simulink model "SSIV_Simulink_Com2"  (R2018a)
settings: Solver=FixedStepAuto  StartTime=0.0  StopTime=inf  FixedStep=.015  RelTol=1e-3  EnableMultiTasking=on
libraries: hdlsllib x51, raspberrypilib x16, simulink x10
(part 1 of 2)
settings Model: SimulationMode=external  Creator=domin  LastModifiedBy=cbirdson
settings SolverCC: ConcurrentTasks=on  PositivePriorityOrder=on  AutoInsertRateTranBlk=on
settings DataIOCC: SaveFormat=Array
settings OptimizationCC: EnhancedBackFolding=on  PassReuseOutputArgsThreshold=0  MaxStackSize=64  OptimizeBlockOrder=speed  DifferentSizesBufferReuse=on  OptimizationCustomize=off
settings DebuggingCC: ParameterTunabilityLossMsg=error
settings HardwareCC: ProdBitPerPointer=32  ProdBitPerSizeT=32  ProdBitPerPtrDiffT=32  ProdLargestAtomicInteger=Long  ProdLargestAtomicFloat=Double  ProdWordSize=32  ProdHWDeviceType=ARM Compatible->ARM Cortex  UseEmbeddedCoderFeatures=off  UseSimulinkCoderFeatures=off
settings SFSimCC: MATLABDynamicMemAlloc=off
settings RTWCC: SystemTargetFile=ert.tlc  HardwareBoard=Raspberry Pi  TLCOptions="-aInlineSetEventsForThisBaseRateFcn=TLC_FALSE -aSuppressMultiTaskScheduler=TLC_FALSE  -aRateBasedStepFcn=0"  TemplateMakefile=ert_default_tmf  RTWVerbose=off  Toolchain=GNU GCC Raspberry Pi  BuildConfiguration=Faster Runs
settings CodeAppCC: ForceParamTrailComments=on  OperatorAnnotations=on  MangleLength=10
settings ERTTargetCC: ERTCustomFileBanners=off  SupportContinuousTime=on  SupportNonInlinedSFcns=on  RemoveResetFunc=off  SupportVariableSizeSignals=on  ModelStepFunctionPrototypeControlCompliant=off  ExtMode=on  ExtModeMexArgs='129.65.101.12' 0 17725  ERTSrcFileBannerTemplate=codertarget_code_template.cgt  ERTHdrFileBannerTemplate=codertarget_code_template.cgt  ERTDataSrcFileTemplate=codertarget_code_template.cgt  ERTDataHdrFileTemplate=codertarget_code_template.cgt

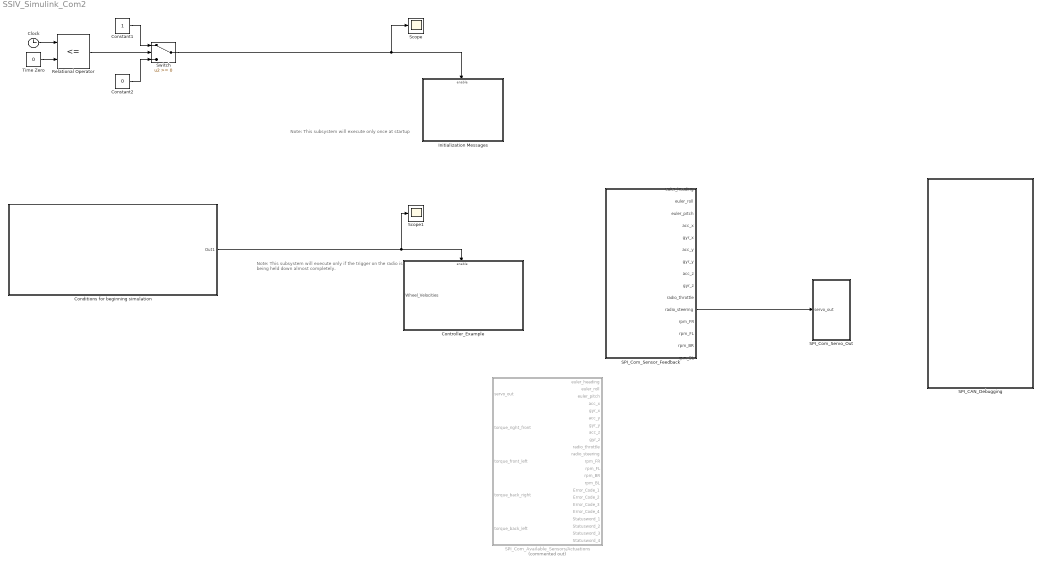
== system SSIV_Simulink_Com2 ==
  note: Note: This subsystem will execute only once at startup
  note: Note: This subsystem will execute only if the trigger on the radio
      | is being held down almost completely.
  Clock : Clock
  Conditions for beginning simulation : Subsystem
  Constant1 : Constant
  Constant2 : Constant  Value=0
  Controller_Example : Subsystem
  Initialization Messages : Subsystem
  Relational Operator : RelationalOperator  Operator=<=  OutDataTypeStr=boolean  RndMeth=Simplest
  SPI_CAN_Debugging : Subsystem
  SPI_Com_Available_Sensors/Actuations : Subsystem  Commented=on
  SPI_Com_Sensor_Feedback : Subsystem
  SPI_Com_Servo_Out : Subsystem
  Scope : Scope
  Scope1 : Scope
  Switch : Switch
  Time Zero : Constant  Value=0
  wires:
  Relational Operator/1 -> Switch/2
  Time Zero/1 -> Relational Operator/2
  Constant2/1 -> Switch/3
  Clock/1 -> Relational Operator/1
  Switch/1 -> Initialization Messages/Enable, Scope/1
  Constant1/1 -> Switch/1
  Conditions for beginning simulation/1(Out1) -> Controller_Example/Enable, Scope1/1
  SPI_Com_Sensor_Feedback/11(radio_steering) -> SPI_Com_Servo_Out/1(servo_out)

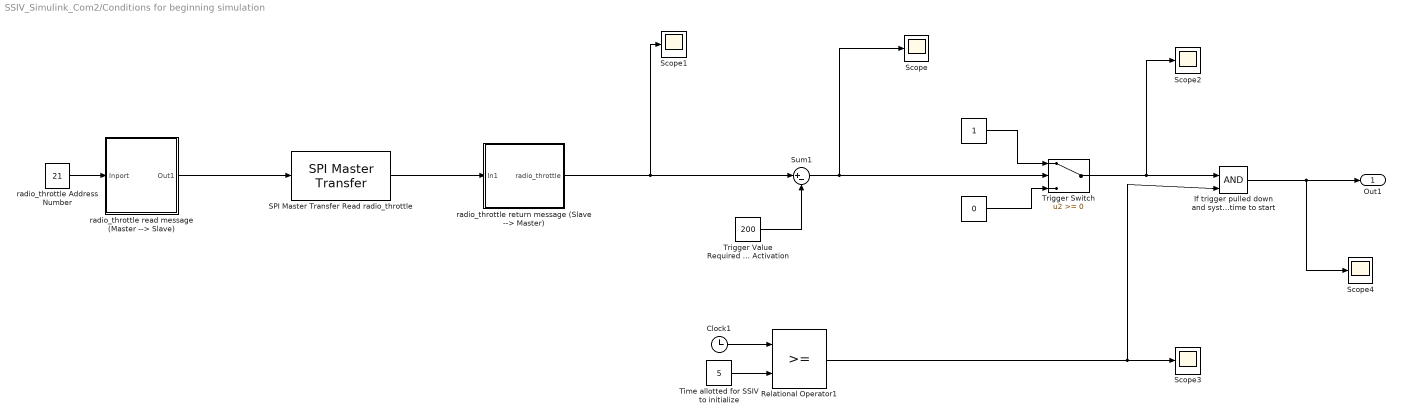
== system SSIV_Simulink_Com2/Conditions for beginning simulation ==
  " " : Constant  Value=0
  "   " : Constant
  Clock1 : Clock
  If trigger pulled down and system given enough time to start : Logic  IconShape=distinctive  AllPortsSameDT=off  OutDataTypeStr=boolean
  Relational Operator1 : RelationalOperator  OutDataTypeStr=boolean  RndMeth=Simplest
  SPI Master Transfer Read radio_throttle : raspberrypilib/SPI Master Transfer  BoardProperty=Pi 3 Model B  SPIModule=uint32(0)  Mode=Master  BusSpeed=1000000  Pin=SPI0_CE1  FirstBitToTransfer=Most significant bit (MSB)  ClockMode=0  BlockFunction=Transfer  RegisterAddress=0  OutputDataType=int8  OutputDataLength=1
      settings: SourceProductName=Simulink Support Package for Raspberry Pi Hardware  SourceProductBaseCode=RASPPI
  Scope{,1..4} (5 alike) : Scope
  Sum1 : Sum  Inputs=|+-
  Time allotted for SSIV to initialize : Constant  Value=5
  Trigger Switch : Switch
  Trigger Value Required for Subsystem Activation : Constant  Value=200
  "radio_throttle Address Number " : Constant  Value=21  OutDataTypeStr=uint8
  radio_throttle read message (Master --> Slave) : Subsystem
  radio_throttle return message (Slave --> Master) : Subsystem
  Out1 : Outport
  wires:
  " "/1 -> Trigger Switch/3
  Trigger Switch/1 -> Scope2/1, If trigger pulled down and system given enough time to start/1
  SPI Master Transfer Read radio_throttle/1 -> radio_throttle return message (Slave --> Master)/1(In1)
  Time allotted for SSIV to initialize/1 -> Relational Operator1/2
  "radio_throttle Address Number "/1 -> radio_throttle read message (Master --> Slave)/1(Inport)
  Clock1/1 -> Relational Operator1/1
  Relational Operator1/1 -> Scope3/1, If trigger pulled down and system given enough time to start/2
  Sum1/1 -> Scope/1, Trigger Switch/2
  radio_throttle read message (Master --> Slave)/1(Out1) -> SPI Master Transfer Read radio_throttle/1
  Trigger Value Required for Subsystem Activation/1 -> Sum1/2
  "   "/1 -> Trigger Switch/1
  If trigger pulled down and system given enough time to start/1 -> Scope4/1, Out1/1
  radio_throttle return message (Slave --> Master)/1(radio_throttle) -> Scope1/1, Sum1/1

== system SSIV_Simulink_Com2/Controller_Example ==
  "Wheel_Velocities " : Inport
  Enable : EnablePort
  Const Mot Torque mNm : Constant  Value=100
  Const Mot Torque mNm1 : Constant  Value=100
  Gain : Gain
  Gain1 : Gain
  SPI_Communication_Torque_Actuations : Subsystem
  wires:
  Const Mot Torque mNm/1 -> Gain/1
  Const Mot Torque mNm1/1 -> Gain1/1
  Gain/1 -> SPI_Communication_Torque_Actuations/2(torque_front_left), SPI_Communication_Torque_Actuations/1(torque_right_front)
  Gain1/1 -> SPI_Communication_Torque_Actuations/4(torque_back_left), SPI_Communication_Torque_Actuations/3(torque_back_right)

== system SSIV_Simulink_Com2/Initialization Messages ==
  Enable : EnablePort
  Dead Switch : Constant  OutDataTypeStr=uint8
  Display3 : Display
      settings: Format=decimal (Stored Integer)
  Display4 : Display
      settings: Format=decimal (Stored Integer)
  Display5 : Display
      settings: Format=decimal (Stored Integer)
  IMU Reset : Constant  OutDataTypeStr=uint8
  Initialize Motor Controllers Command : Constant  OutDataTypeStr=uint8
  SPI Register Write dead_switch : raspberrypilib/SPI Register Write  BoardProperty=Pi 3 Model B  SPIModule=uint32(0)  Mode=Master  BusSpeed=1000000  Pin=SPI0_CE1  FirstBitToTransfer=Most significant bit (MSB)  ClockMode=0  BlockFunction=Write  RegisterAddress=2  OutputDataType=int8  OutputDataLength=1
      settings: SourceProductName=Simulink Support Package for Raspberry Pi Hardware  SourceProductBaseCode=RASPPI
  SPI Register Write init_motor_controllers : raspberrypilib/SPI Register Write  BoardProperty=Pi 3 Model B  SPIModule=uint32(0)  Mode=Master  BusSpeed=1000000  Pin=SPI0_CE1  FirstBitToTransfer=Most significant bit (MSB)  ClockMode=0  BlockFunction=Write  RegisterAddress=0  OutputDataType=int8  OutputDataLength=1
      settings: SourceProductName=Simulink Support Package for Raspberry Pi Hardware  SourceProductBaseCode=RASPPI
  SPI Register Write reset_imu : raspberrypilib/SPI Register Write  BoardProperty=Pi 3 Model B  SPIModule=uint32(0)  Mode=Master  BusSpeed=1000000  Pin=SPI0_CE1  FirstBitToTransfer=Most significant bit (MSB)  ClockMode=0  BlockFunction=Write  RegisterAddress=1  OutputDataType=int8  OutputDataLength=1
      settings: SourceProductName=Simulink Support Package for Raspberry Pi Hardware  SourceProductBaseCode=RASPPI
  wires:
  Initialize Motor Controllers Command/1 -> Display3/1, SPI Register Write init_motor_controllers/1
  IMU Reset/1 -> SPI Register Write reset_imu/1, Display4/1
  Dead Switch/1 -> Display5/1, SPI Register Write dead_switch/1

== system SSIV_Simulink_Com2/SPI_CAN_Debugging ==
  Bitwise AND : simulink/Logic and Bit Operations/Bitwise Operator  logicop=AND  UseBitMask=on  BitMask=bin2dec('01101111')  BitMaskRealWorld=Stored Integer
  Debugging : Scope  NumInputPorts=2
  ERROR_REGISTERS : Display
      settings: Format=binary (Stored Integer)
  Error and Statusword read message (Master --> Slave) : Subsystem
  Errors and Statuswords return message (Slave --> Master) : Subsystem
  Mux : Mux
  Mux1 : Mux
  SPI Master Transfer Read Errors and Statuswords : raspberrypilib/SPI Master Transfer  BoardProperty=Pi 3 Model B  SPIModule=uint32(0)  Mode=Master  BusSpeed=1000000  Pin=SPI0_CE1  FirstBitToTransfer=Most significant bit (MSB)  ClockMode=0  BlockFunction=Transfer  RegisterAddress=0  OutputDataType=int8  OutputDataLength=1
      settings: SourceProductName=Simulink Support Package for Raspberry Pi Hardware  SourceProductBaseCode=RASPPI
  STATUSWORDS : Display
      settings: Format=binary (Stored Integer)
  node_errors[0] Address Number : Constant  Value=44  OutDataTypeStr=uint8
  wires:
  Error and Statusword read message (Master --> Slave)/1(Out1) -> SPI Master Transfer Read Errors and Statuswords/1
  node_errors[0] Address Number/1 -> Error and Statusword read message (Master --> Slave)/1(Inport)
  SPI Master Transfer Read Errors and Statuswords/1 -> Bitwise AND/1
  Bitwise AND/1 -> Errors and Statuswords return message (Slave --> Master)/1(In1)
  Errors and Statuswords return message (Slave --> Master)/1(Error_Code_1) -> Mux/1
  Errors and Statuswords return message (Slave --> Master)/2(Error_Code_2) -> Mux/2
  Errors and Statuswords return message (Slave --> Master)/3(Error_Code_3) -> Mux/3
  Errors and Statuswords return message (Slave --> Master)/4(Error_Code_4) -> Mux/4
  Mux/1 -> ERROR_REGISTERS/1, Debugging/1
  Errors and Statuswords return message (Slave --> Master)/5(Statusword_1) -> Mux1/1
  Errors and Statuswords return message (Slave --> Master)/6(Statusword_2) -> Mux1/2
  Errors and Statuswords return message (Slave --> Master)/7(Statusword_3) -> Mux1/3
  Errors and Statuswords return message (Slave --> Master)/8(Statusword_4) -> Mux1/4
  Mux1/1 -> STATUSWORDS/1, Debugging/2

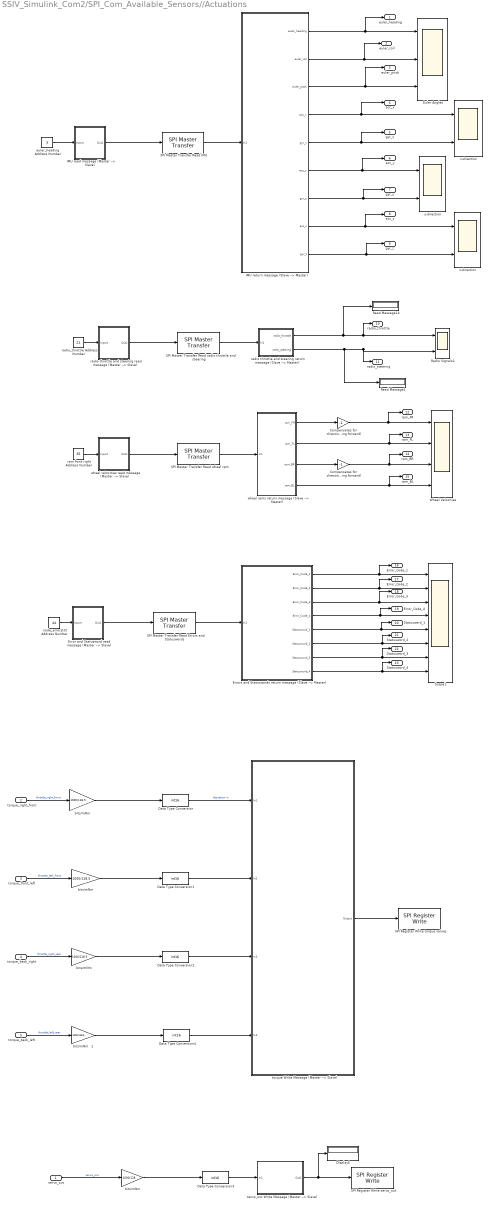
== system SSIV_Simulink_Com2/SPI_Com_Available_Sensors//Actuations ==
  servo_out : Inport
  torque_right_front : Inport  Port=2
  torque_front_left : Inport  Port=3
  torque_back_right : Inport  Port=4
  torque_back_left : Inport  Port=5
  Compensates for direction of spin (want positive to be rolling forward) : Gain  Gain=-1
  "Compensates for direction of spin (want positive to be rolling forward)  " : Gain  Gain=-1
  Data Type Conversion{,1..4} (5 alike) : DataTypeConversion  OutDataTypeStr=int16  RndMeth=Nearest
  Display5 : Display
      settings: Format=decimal (Stored Integer)
  Error and Statusword read message (Master --> Slave) : Subsystem
  Errors and Statuswords return message (Slave --> Master) : Subsystem
  Euler Angles : Scope  NumInputPorts=3
  IMU read message (Master --> Slave) : Subsystem
  IMU return message (Slave --> Master) : Subsystem
  Radio SIgnals2 : Scope  NumInputPorts=2
  Read Message1 : Display
      settings: Format=decimal (Stored Integer)
  Read Message14 : Display
      settings: Format=decimal (Stored Integer)
  SPI Master Transfer Read Errors and Statuswords : raspberrypilib/SPI Master Transfer  BoardProperty=Pi 3 Model B  SPIModule=uint32(0)  Mode=Master  BusSpeed=1000000  Pin=SPI0_CE1  FirstBitToTransfer=Most significant bit (MSB)  ClockMode=0  BlockFunction=Transfer  RegisterAddress=0  OutputDataType=int8  OutputDataLength=1
      settings: SourceProductName=Simulink Support Package for Raspberry Pi Hardware  SourceProductBaseCode=RASPPI
  SPI Master Transfer Read IMU : raspberrypilib/SPI Master Transfer  BoardProperty=Pi 3 Model B  SPIModule=uint32(0)  Mode=Master  BusSpeed=1000000  Pin=SPI0_CE1  FirstBitToTransfer=Most significant bit (MSB)  ClockMode=0  BlockFunction=Transfer  RegisterAddress=0  OutputDataType=int8  OutputDataLength=1
      settings: SourceProductName=Simulink Support Package for Raspberry Pi Hardware  SourceProductBaseCode=RASPPI
  SPI Master Transfer Read radio throttle and steering : raspberrypilib/SPI Master Transfer  BoardProperty=Pi 3 Model B  SPIModule=uint32(0)  Mode=Master  BusSpeed=1000000  Pin=SPI0_CE1  FirstBitToTransfer=Most significant bit (MSB)  ClockMode=0  BlockFunction=Transfer  RegisterAddress=0  OutputDataType=int8  OutputDataLength=1
      settings: SourceProductName=Simulink Support Package for Raspberry Pi Hardware  SourceProductBaseCode=RASPPI
  SPI Master Transfer Read wheel rpm : raspberrypilib/SPI Master Transfer  BoardProperty=Pi 3 Model B  SPIModule=uint32(0)  Mode=Master  BusSpeed=1000000  Pin=SPI0_CE1  FirstBitToTransfer=Most significant bit (MSB)  ClockMode=0  BlockFunction=Transfer  RegisterAddress=0  OutputDataType=int8  OutputDataLength=1
      settings: SourceProductName=Simulink Support Package for Raspberry Pi Hardware  SourceProductBaseCode=RASPPI
  "SPI Register Write servo_out " : raspberrypilib/SPI Register Write  BoardProperty=Pi 3 Model B  SPIModule=uint32(0)  Mode=Master  BusSpeed=1000000  Pin=SPI0_CE1  FirstBitToTransfer=Most significant bit (MSB)  ClockMode=0  BlockFunction=Write  RegisterAddress=33  OutputDataType=int8  OutputDataLength=1
      settings: SourceProductName=Simulink Support Package for Raspberry Pi Hardware  SourceProductBaseCode=RASPPI
  SPI Register Write torque values : raspberrypilib/SPI Register Write  BoardProperty=Pi 3 Model B  SPIModule=uint32(0)  Mode=Master  BusSpeed=1000000  Pin=SPI0_CE1  FirstBitToTransfer=Most significant bit (MSB)  ClockMode=0  BlockFunction=Write  RegisterAddress=25  OutputDataType=int8  OutputDataLength=1
      settings: SourceProductName=Simulink Support Package for Raspberry Pi Hardware  SourceProductBaseCode=RASPPI
  Scope1 : Scope  NumInputPorts=8
  Wheel Velocities : Scope  NumInputPorts=4
  bits/mNm : Gain  Gain=1000/118.5
  "bits/mNm " : Gain  Gain=1000/118.5
  "bits/mNm  " : Gain  Gain=1000/118.5
  "bits/mNm    " : Gain  Gain=1000/128
  bits/mNm   1 : Gain  Gain=1000/118.5
  euler_heading Address Number : Constant  Value=3  OutDataTypeStr=uint8
  node_errors[0] Address Number : Constant  Value=44  OutDataTypeStr=uint8
  radio throttle and steering read message (Master --> Slave) : Subsystem
  radio throttle and steering return message (Slave --> Master) : Subsystem
  "radio_throttle Address Number " : Constant  Value=21  OutDataTypeStr=uint8
  "rpm front right Address Number " : Constant  Value=35  OutDataTypeStr=uint8
  servo_out Write Message (Master --> Slave) : Subsystem
  torque Write Message (Master --> Slave) : Subsystem
  wheel rpms return message (Slave --> Master) : Subsystem
  wheel velocities read message (Master --> Slave) : Subsystem
  x-direction : Scope  NumInputPorts=2
  y-direction : Scope  NumInputPorts=2
  z-direction : Scope  NumInputPorts=2
  euler_heading : Outport
  euler_roll : Outport  Port=2
  euler_pitch : Outport  Port=3
  acc_x : Outport  Port=4
  gyr_x : Outport  Port=5
  acc_y : Outport  Port=6
  gyr_y : Outport  Port=7
  acc_z : Outport  Port=8
  gyr_z : Outport  Port=9
  radio_throttle : Outport  Port=10
  radio_steering : Outport  Port=11
  rpm_FR : Outport  Port=12
  rpm_FL : Outport  Port=13
  rpm_BR : Outport  Port=14
  rpm_BL : Outport  Port=15
  Error_Code_1 : Outport  Port=16
  Error_Code_2 : Outport  Port=17
  Error_Code_3 : Outport  Port=18
  Error_Code_4 : Outport  Port=19
  Statusword_1 : Outport  Port=20
  Statusword_2 : Outport  Port=21
  Statusword_3 : Outport  Port=22
  Statusword_4 : Outport  Port=23
  wires:
  IMU read message (Master --> Slave)/1(Out1) -> SPI Master Transfer Read IMU/1
  SPI Master Transfer Read IMU/1 -> IMU return message (Slave --> Master)/1(In1)
  SPI Master Transfer Read wheel rpm/1 -> wheel rpms return message (Slave --> Master)/1(In1)
  wheel rpms return message (Slave --> Master)/1(rpm_FR) -> Compensates for direction of spin (want positive to be rolling forward)/1
  servo_out/1 -> "bits/mNm    "/1  "servo_out"
  servo_out Write Message (Master --> Slave)/1(Out1) -> Display5/1, "SPI Register Write servo_out "/1
  torque Write Message (Master --> Slave)/1(Output) -> SPI Register Write torque values/1
  Data Type Conversion/1 -> torque Write Message (Master --> Slave)/1(In1)  "Actuation in"
  Data Type Conversion1/1 -> torque Write Message (Master --> Slave)/2(In2)
  Data Type Conversion2/1 -> torque Write Message (Master --> Slave)/3(In3)
  Data Type Conversion3/1 -> servo_out Write Message (Master --> Slave)/1(In1)
  Data Type Conversion4/1 -> torque Write Message (Master --> Slave)/4(In4)
  euler_heading Address Number/1 -> IMU read message (Master --> Slave)/1(Inport)
  "radio_throttle Address Number "/1 -> radio throttle and steering read message (Master --> Slave)/1(Inport)
  radio throttle and steering return message (Slave --> Master)/1(radio_throttle) -> Radio SIgnals2/1, radio_throttle/1, Read Message14/1
  SPI Master Transfer Read radio throttle and steering/1 -> radio throttle and steering return message (Slave --> Master)/1(In1)
  radio throttle and steering read message (Master --> Slave)/1(Out1) -> SPI Master Transfer Read radio throttle and steering/1
  bits/mNm/1 -> Data Type Conversion/1
  "bits/mNm "/1 -> Data Type Conversion1/1
  "bits/mNm  "/1 -> Data Type Conversion2/1
  bits/mNm   1/1 -> Data Type Conversion4/1
  "bits/mNm    "/1 -> Data Type Conversion3/1
  Compensates for direction of spin (want positive to be rolling forward)/1 -> Wheel Velocities/1, rpm_FR/1
  Error and Statusword read message (Master --> Slave)/1(Out1) -> SPI Master Transfer Read Errors and Statuswords/1
  SPI Master Transfer Read Errors and Statuswords/1 -> Errors and Statuswords return message (Slave --> Master)/1(In1)
  node_errors[0] Address Number/1 -> Error and Statusword read message (Master --> Slave)/1(Inport)
  Errors and Statuswords return message (Slave --> Master)/1(Error_Code_1) -> Error_Code_1/1, Scope1/1
  Errors and Statuswords return message (Slave --> Master)/2(Error_Code_2) -> Error_Code_2/1, Scope1/2
  Errors and Statuswords return message (Slave --> Master)/3(Error_Code_3) -> Error_Code_3/1, Scope1/3
  Errors and Statuswords return message (Slave --> Master)/4(Error_Code_4) -> Error_Code_4/1, Scope1/4
  Errors and Statuswords return message (Slave --> Master)/5(Statusword_1) -> Statusword_1/1, Scope1/5
  Errors and Statuswords return message (Slave --> Master)/6(Statusword_2) -> Statusword_2/1, Scope1/6
  Errors and Statuswords return message (Slave --> Master)/7(Statusword_3) -> Statusword_3/1, Scope1/7
  Errors and Statuswords return message (Slave --> Master)/8(Statusword_4) -> Statusword_4/1, Scope1/8
  "rpm front right Address Number "/1 -> wheel velocities read message (Master --> Slave)/1(Inport)
  wheel velocities read message (Master --> Slave)/1(Out1) -> SPI Master Transfer Read wheel rpm/1
  wheel rpms return message (Slave --> Master)/2(rpm_FL) -> rpm_FL/1, Wheel Velocities/2
  wheel rpms return message (Slave --> Master)/3(rpm_BR) -> "Compensates for direction of spin (want positive to be rolling forward)  "/1
  "Compensates for direction of spin (want positive to be rolling forward)  "/1 -> rpm_BR/1, Wheel Velocities/3
  wheel rpms return message (Slave --> Master)/4(rpm_BL) -> rpm_BL/1, Wheel Velocities/4
  radio throttle and steering return message (Slave --> Master)/2(radio_steering) -> Read Message1/1, radio_steering/1, Radio SIgnals2/2
  IMU return message (Slave --> Master)/1(euler_heading) -> euler_heading/1, Euler Angles/1
  IMU return message (Slave --> Master)/2(euler_roll) -> euler_roll/1, Euler Angles/2
  IMU return message (Slave --> Master)/3(euler_pitch) -> euler_pitch/1, Euler Angles/3
  IMU return message (Slave --> Master)/4(acc_x) -> acc_x/1, x-direction/1
  IMU return message (Slave --> Master)/5(gyr_x) -> gyr_x/1, x-direction/2
  IMU return message (Slave --> Master)/6(acc_y) -> acc_y/1, y-direction/1
  IMU return message (Slave --> Master)/7(gyr_y) -> gyr_y/1, y-direction/2
  IMU return message (Slave --> Master)/8(acc_z) -> acc_z/1, z-direction/1
  IMU return message (Slave --> Master)/9(gyr_z) -> gyr_z/1, z-direction/2
  torque_back_left/1 -> bits/mNm   1/1  "throttle_left_rear"
  torque_right_front/1 -> bits/mNm/1  "throttle_right_front"
  torque_front_left/1 -> "bits/mNm "/1  "throttle_left_front"
  torque_back_right/1 -> "bits/mNm  "/1  "throttle_right_rear"

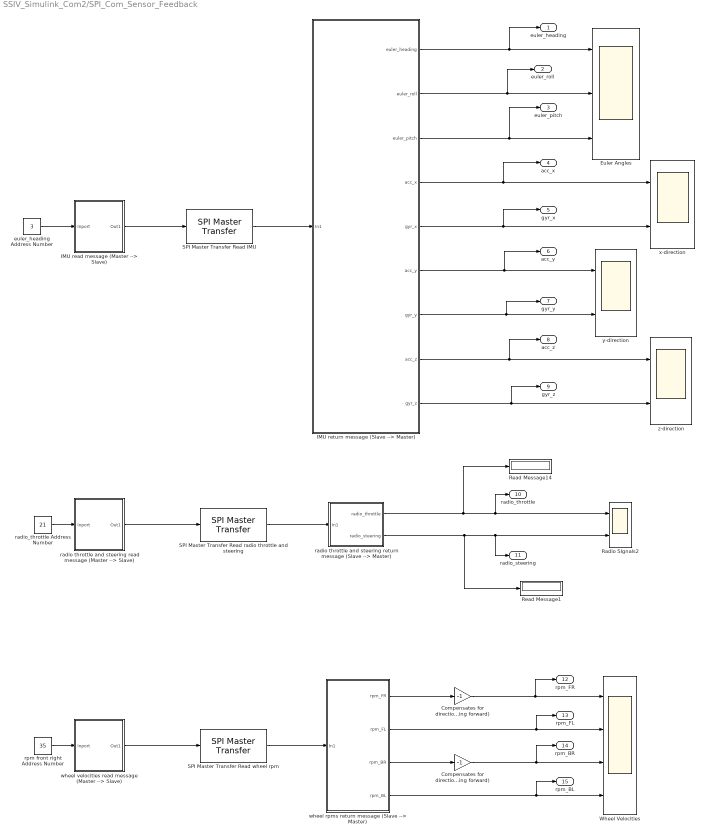
== system SSIV_Simulink_Com2/SPI_Com_Sensor_Feedback ==
  Compensates for direction of spin (want positive to be rolling forward) : Gain  Gain=-1
  "Compensates for direction of spin (want positive to be rolling forward)  " : Gain  Gain=-1
  Euler Angles : Scope  NumInputPorts=3
  IMU read message (Master --> Slave) : Subsystem
  IMU return message (Slave --> Master) : Subsystem
  Radio SIgnals2 : Scope  NumInputPorts=2
  Read Message1 : Display
      settings: Format=decimal (Stored Integer)
  Read Message14 : Display
      settings: Format=decimal (Stored Integer)
  SPI Master Transfer Read IMU : raspberrypilib/SPI Master Transfer  BoardProperty=Pi 3 Model B  SPIModule=uint32(0)  Mode=Master  BusSpeed=1000000  Pin=SPI0_CE1  FirstBitToTransfer=Most significant bit (MSB)  ClockMode=0  BlockFunction=Transfer  RegisterAddress=0  OutputDataType=int8  OutputDataLength=1
      settings: SourceProductName=Simulink Support Package for Raspberry Pi Hardware  SourceProductBaseCode=RASPPI
  SPI Master Transfer Read radio throttle and steering : raspberrypilib/SPI Master Transfer  BoardProperty=Pi 3 Model B  SPIModule=uint32(0)  Mode=Master  BusSpeed=1000000  Pin=SPI0_CE1  FirstBitToTransfer=Most significant bit (MSB)  ClockMode=0  BlockFunction=Transfer  RegisterAddress=0  OutputDataType=int8  OutputDataLength=1
      settings: SourceProductName=Simulink Support Package for Raspberry Pi Hardware  SourceProductBaseCode=RASPPI
  SPI Master Transfer Read wheel rpm : raspberrypilib/SPI Master Transfer  BoardProperty=Pi 3 Model B  SPIModule=uint32(0)  Mode=Master  BusSpeed=1000000  Pin=SPI0_CE1  FirstBitToTransfer=Most significant bit (MSB)  ClockMode=0  BlockFunction=Transfer  RegisterAddress=0  OutputDataType=int8  OutputDataLength=1
      settings: SourceProductName=Simulink Support Package for Raspberry Pi Hardware  SourceProductBaseCode=RASPPI
  Wheel Velocities : Scope  NumInputPorts=4
  euler_heading Address Number : Constant  Value=3  OutDataTypeStr=uint8
  radio throttle and steering read message (Master --> Slave) : Subsystem
  radio throttle and steering return message (Slave --> Master) : Subsystem
  "radio_throttle Address Number " : Constant  Value=21  OutDataTypeStr=uint8
  "rpm front right Address Number " : Constant  Value=35  OutDataTypeStr=uint8
  wheel rpms return message (Slave --> Master) : Subsystem
  wheel velocities read message (Master --> Slave) : Subsystem
  x-direction : Scope  NumInputPorts=2
  y-direction : Scope  NumInputPorts=2
  z-direction : Scope  NumInputPorts=2
  euler_heading : Outport
  euler_roll : Outport  Port=2
  euler_pitch : Outport  Port=3
  acc_x : Outport  Port=4
  gyr_x : Outport  Port=5
  acc_y : Outport  Port=6
  gyr_y : Outport  Port=7
  acc_z : Outport  Port=8
  gyr_z : Outport  Port=9
  radio_throttle : Outport  Port=10
  radio_steering : Outport  Port=11
  rpm_FR : Outport  Port=12
  rpm_FL : Outport  Port=13
  rpm_BR : Outport  Port=14
  rpm_BL : Outport  Port=15
  wires:
  SPI Master Transfer Read radio throttle and steering/1 -> radio throttle and steering return message (Slave --> Master)/1(In1)
  radio throttle and steering read message (Master --> Slave)/1(Out1) -> SPI Master Transfer Read radio throttle and steering/1
  euler_heading Address Number/1 -> IMU read message (Master --> Slave)/1(Inport)
  "radio_throttle Address Number "/1 -> radio throttle and steering read message (Master --> Slave)/1(Inport)
  radio throttle and steering return message (Slave --> Master)/1(radio_throttle) -> Radio SIgnals2/1, radio_throttle/1, Read Message14/1
  IMU read message (Master --> Slave)/1(Out1) -> SPI Master Transfer Read IMU/1
  SPI Master Transfer Read IMU/1 -> IMU return message (Slave --> Master)/1(In1)
  IMU return message (Slave --> Master)/1(euler_heading) -> euler_heading/1, Euler Angles/1
  IMU return message (Slave --> Master)/8(acc_z) -> acc_z/1, z-direction/1
  IMU return message (Slave --> Master)/6(acc_y) -> acc_y/1, y-direction/1
  IMU return message (Slave --> Master)/9(gyr_z) -> gyr_z/1, z-direction/2
  IMU return message (Slave --> Master)/5(gyr_x) -> gyr_x/1, x-direction/2
  IMU return message (Slave --> Master)/3(euler_pitch) -> euler_pitch/1, Euler Angles/3
  IMU return message (Slave --> Master)/2(euler_roll) -> euler_roll/1, Euler Angles/2
  radio throttle and steering return message (Slave --> Master)/2(radio_steering) -> Read Message1/1, radio_steering/1, Radio SIgnals2/2
  IMU return message (Slave --> Master)/4(acc_x) -> acc_x/1, x-direction/1
  IMU return message (Slave --> Master)/7(gyr_y) -> gyr_y/1, y-direction/2
  wheel rpms return message (Slave --> Master)/3(rpm_BR) -> "Compensates for direction of spin (want positive to be rolling forward)  "/1
  "Compensates for direction of spin (want positive to be rolling forward)  "/1 -> rpm_BR/1, Wheel Velocities/3
  wheel rpms return message (Slave --> Master)/4(rpm_BL) -> rpm_BL/1, Wheel Velocities/4
  "rpm front right Address Number "/1 -> wheel velocities read message (Master --> Slave)/1(Inport)
  wheel velocities read message (Master --> Slave)/1(Out1) -> SPI Master Transfer Read wheel rpm/1
  wheel rpms return message (Slave --> Master)/2(rpm_FL) -> rpm_FL/1, Wheel Velocities/2
  wheel rpms return message (Slave --> Master)/1(rpm_FR) -> Compensates for direction of spin (want positive to be rolling forward)/1
  Compensates for direction of spin (want positive to be rolling forward)/1 -> Wheel Velocities/1, rpm_FR/1
  SPI Master Transfer Read wheel rpm/1 -> wheel rpms return message (Slave --> Master)/1(In1)

== system SSIV_Simulink_Com2/SPI_Com_Servo_Out ==
  servo_out : Inport
  Data Type Conversion3 : DataTypeConversion  OutDataTypeStr=int16  RndMeth=Nearest
  Display5 : Display
      settings: Format=decimal (Stored Integer)
  "SPI Register Write servo_out " : raspberrypilib/SPI Register Write  BoardProperty=Pi 3 Model B  SPIModule=uint32(0)  Mode=Master  BusSpeed=1000000  Pin=SPI0_CE1  FirstBitToTransfer=Most significant bit (MSB)  ClockMode=0  BlockFunction=Write  RegisterAddress=33  OutputDataType=int8  OutputDataLength=1
      settings: SourceProductName=Simulink Support Package for Raspberry Pi Hardware  SourceProductBaseCode=RASPPI
  servo_out Write Message (Master --> Slave) : Subsystem
  wires:
  Data Type Conversion3/1 -> servo_out Write Message (Master --> Slave)/1(In1)
  servo_out/1 -> Data Type Conversion3/1  "servo_out"
  servo_out Write Message (Master --> Slave)/1(Out1) -> Display5/1, "SPI Register Write servo_out "/1

== system SSIV_Simulink_Com2/Conditions for beginning simulation/radio_throttle read message (Master --> Slave) ==
  Inport : Inport
  Mux : Mux
      settings: DisplayOption=signals
  Read Bit Set : simulink/Logic and Bit Operations/Bit Set  iBit=7
      settings: SourceProductName=Simulink  SourceProductBaseCode=SL
  uint8_t 1 : Constant  OutDataTypeStr=uint8
  uint8_t 2 : Constant  OutDataTypeStr=uint8
  uint8_t 3 : Constant  OutDataTypeStr=uint8
  Out1 : Outport
  wires:
  Read Bit Set/1 -> Mux/1  "Addres/RW Byte radio_throttle Teensy Status will be returned here"
  uint8_t 1/1 -> Mux/2  "Junk will be returned here"
  Inport/1 -> Read Bit Set/1
  uint8_t 3/1 -> Mux/4  "Byte 1 will be returned here"
  Mux/1 -> Out1/1
  uint8_t 2/1 -> Mux/3  "Byte 0 will be returned here"

== system SSIV_Simulink_Com2/Conditions for beginning simulation/radio_throttle return message (Slave --> Master) ==
  In1 : Inport
  8 bytes concatinated converted to double : DataTypeConversion  OutDataTypeStr=double  RndMeth=Nearest
  Bit Concat : hdlsllib/Logic and Bit Operations/Bit Concat  numInputs=2
      settings: SourceProductName=HDL Coder  SourceProductBaseCode=HD
  Bytes of the return message : Display
      settings: Format=decimal (Stored Integer)
  Data Type Conversion : DataTypeConversion  OutDataTypeStr=int16  RndMeth=Nearest
  Demux : Demux
  Display : Display
      settings: Format=binary (Stored Integer)
  Display1 : Display
      settings: Format=decimal (Stored Integer)
  Display2 : Display
      settings: Format=binary (Stored Integer)
  radio_throttle : Outport
  wires:
  8 bytes concatinated converted to double/1 -> Display1/1, radio_throttle/1  "radio_throttle"
  Demux/2 -> Display2/1  "Slave Status"
  Demux/1 -> Display/1  "Previous Data"
  In1/1 -> Bytes of the return message/1, Demux/1
  Bit Concat/1 -> Data Type Conversion/1
  Demux/4 -> Bit Concat/1
  Demux/3 -> Bit Concat/2
  Data Type Conversion/1 -> 8 bytes concatinated converted to double/1

== system SSIV_Simulink_Com2/Controller_Example/SPI_Communication_Torque_Actuations ==
  torque_right_front : Inport
  torque_front_left : Inport  Port=2
  torque_back_right : Inport  Port=3
  torque_back_left : Inport  Port=4
  Data Type Conversion{4..7} (4 alike) : DataTypeConversion  OutDataTypeStr=int16  RndMeth=Nearest
  SPI Register Write torque values : raspberrypilib/SPI Register Write  BoardProperty=Pi 3 Model B  SPIModule=uint32(0)  Mode=Master  BusSpeed=1000000  Pin=SPI0_CE1  FirstBitToTransfer=Most significant bit (MSB)  ClockMode=0  BlockFunction=Write  RegisterAddress=25  OutputDataType=int8  OutputDataLength=1
      settings: SourceProductName=Simulink Support Package for Raspberry Pi Hardware  SourceProductBaseCode=RASPPI
  bits/mNm   2 : Gain  Gain=1000/118.5
  bits/mNm  1 : Gain  Gain=1000/118.5
  bits/mNm 1 : Gain  Gain=1000/118.5
  bits/mNm1 : Gain  Gain=1000/118.5
  torque Write Message (Master --> Slave) : Subsystem
  wires:
  Data Type Conversion4/1 -> torque Write Message (Master --> Slave)/1(In1)
  torque_back_right/1 -> bits/mNm  1/1  "throttle_right_rear"
  torque_front_left/1 -> bits/mNm 1/1  "throttle_left_front"
  torque_back_left/1 -> bits/mNm   2/1  "throttle_left_rear"
  torque_right_front/1 -> bits/mNm1/1  "throttle_right_front"
  bits/mNm 1/1 -> Data Type Conversion5/1
  Data Type Conversion7/1 -> torque Write Message (Master --> Slave)/4(In4)
  bits/mNm  1/1 -> Data Type Conversion6/1
  Data Type Conversion5/1 -> torque Write Message (Master --> Slave)/2(In2)
  torque Write Message (Master --> Slave)/1(Output) -> SPI Register Write torque values/1
  bits/mNm1/1 -> Data Type Conversion4/1
  Data Type Conversion6/1 -> torque Write Message (Master --> Slave)/3(In3)
  bits/mNm   2/1 -> Data Type Conversion7/1

== system SSIV_Simulink_Com2/SPI_CAN_Debugging/Error and Statusword read message (Master --> Slave) ==
  Inport : Inport
  Mux : Mux  Inputs=10
      settings: DisplayOption=signals
  Read Bit Set : simulink/Logic and Bit Operations/Bit Set  iBit=7
      settings: SourceProductName=Simulink  SourceProductBaseCode=SL
  uint8_t {1..9} (9 alike) : Constant  OutDataTypeStr=uint8
  Out1 : Outport
  wires:
  Read Bit Set/1 -> Mux/1  "Addres/RW Byte velocity_RL Teensy Status will be returned here"
  uint8_t 1/1 -> Mux/2  "Junk will be returned here"
  Inport/1 -> Read Bit Set/1
  uint8_t 3/1 -> Mux/4  "Byte 1 will be returned here"
  Mux/1 -> Out1/1
  uint8_t 2/1 -> Mux/3  "Byte 0 will be returned here"
  uint8_t 5/1 -> Mux/6  "Byte 3 will be returned here"
  uint8_t 6/1 -> Mux/7  "Byte 4 will be returned here"
  uint8_t 4/1 -> Mux/5  "Byte 2 will be returned here"
  uint8_t 8/1 -> Mux/9  "Byte 6 will be returned here"
  uint8_t 7/1 -> Mux/8  "Byte 5  will be returned here"
  uint8_t 9/1 -> Mux/10  "Byte 7 will be returned here"

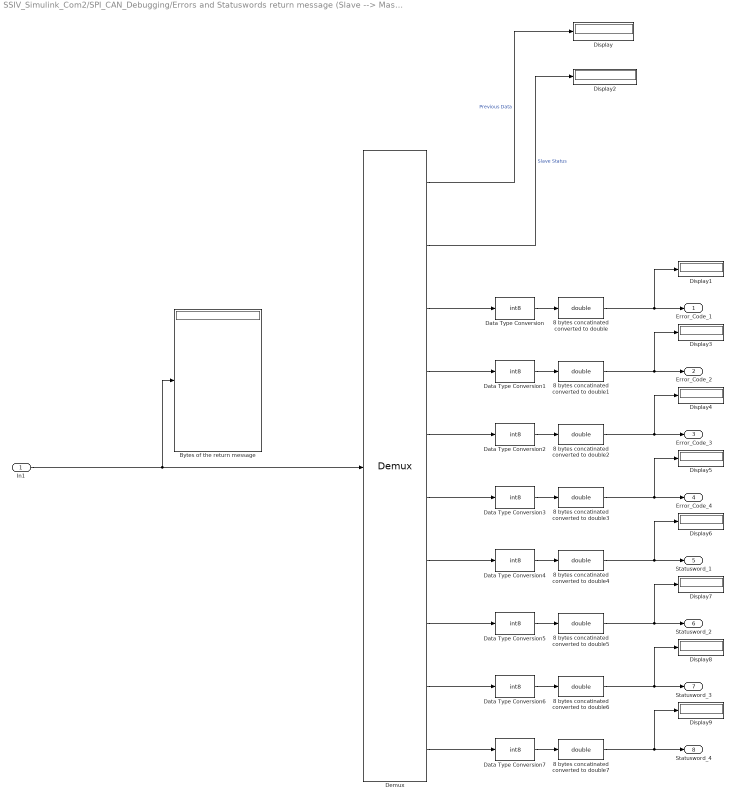
== system SSIV_Simulink_Com2/SPI_CAN_Debugging/Errors and Statuswords return message (Slave --> Master) ==
  In1 : Inport
  8 bytes concatinated converted to double{,1..7} (8 alike) : DataTypeConversion  OutDataTypeStr=double  RndMeth=Nearest
  Bytes of the return message : Display
      settings: Format=decimal (Stored Integer)
  Data Type Conversion{,1..7} (8 alike) : DataTypeConversion  OutDataTypeStr=int8  RndMeth=Nearest
  Demux : Demux  Outputs=10
  Display{,1..9} (10 alike) : Display
      Display settings: Format=binary (Stored Integer)
      Display1 settings: Format=hex (Stored Integer)
      Display2 settings: Format=binary (Stored Integer)
      Display3 settings: Format=hex (Stored Integer)
      Display4 settings: Format=hex (Stored Integer)
      Display5 settings: Format=hex (Stored Integer)
      Display6 settings: Format=hex (Stored Integer)
      Display7 settings: Format=hex (Stored Integer)
      Display8 settings: Format=hex (Stored Integer)
      Display9 settings: Format=hex (Stored Integer)
  Error_Code_1 : Outport
  Error_Code_2 : Outport  Port=2
  Error_Code_3 : Outport  Port=3
  Error_Code_4 : Outport  Port=4
  Statusword_1 : Outport  Port=5
  Statusword_2 : Outport  Port=6
  Statusword_3 : Outport  Port=7
  Statusword_4 : Outport  Port=8
  wires:
  8 bytes concatinated converted to double/1 -> Display1/1, Error_Code_1/1
  Demux/1 -> Display/1  "Previous Data"
  In1/1 -> Bytes of the return message/1, Demux/1
  Data Type Conversion/1 -> 8 bytes concatinated converted to double/1
  Demux/2 -> Display2/1  "Slave Status"
  Demux/3 -> Data Type Conversion/1
  Demux/4 -> Data Type Conversion1/1
  Data Type Conversion1/1 -> 8 bytes concatinated converted to double1/1
  8 bytes concatinated converted to double1/1 -> Error_Code_2/1, Display3/1
  8 bytes concatinated converted to double2/1 -> Display4/1, Error_Code_3/1
  Data Type Conversion2/1 -> 8 bytes concatinated converted to double2/1
  Demux/5 -> Data Type Conversion2/1
  Data Type Conversion3/1 -> 8 bytes concatinated converted to double3/1
  8 bytes concatinated converted to double3/1 -> Error_Code_4/1, Display5/1
  Demux/6 -> Data Type Conversion3/1
  8 bytes concatinated converted to double4/1 -> Display6/1, Statusword_1/1
  Data Type Conversion4/1 -> 8 bytes concatinated converted to double4/1
  Demux/7 -> Data Type Conversion4/1
  Demux/8 -> Data Type Conversion5/1
  Data Type Conversion5/1 -> 8 bytes concatinated converted to double5/1
  8 bytes concatinated converted to double5/1 -> Statusword_2/1, Display7/1
  8 bytes concatinated converted to double6/1 -> Display8/1, Statusword_3/1
  Data Type Conversion6/1 -> 8 bytes concatinated converted to double6/1
  Demux/9 -> Data Type Conversion6/1
  Data Type Conversion7/1 -> 8 bytes concatinated converted to double7/1
  8 bytes concatinated converted to double7/1 -> Statusword_4/1, Display9/1
  Demux/10 -> Data Type Conversion7/1

== system SSIV_Simulink_Com2/SPI_Com_Available_Sensors//Actuations/Error and Statusword read message (Master --> Slave) ==
  Inport : Inport
  Mux : Mux  Inputs=10
      settings: DisplayOption=signals
  Read Bit Set : simulink/Logic and Bit Operations/Bit Set  iBit=7
      settings: SourceProductName=Simulink  SourceProductBaseCode=SL
  uint8_t {1..9} (9 alike) : Constant  OutDataTypeStr=uint8
  Out1 : Outport
  wires:
  Read Bit Set/1 -> Mux/1  "Addres/RW Byte velocity_RL Teensy Status will be returned here"
  uint8_t 1/1 -> Mux/2  "Junk will be returned here"
  Inport/1 -> Read Bit Set/1
  uint8_t 3/1 -> Mux/4  "Byte 1 will be returned here"
  Mux/1 -> Out1/1
  uint8_t 2/1 -> Mux/3  "Byte 0 will be returned here"
  uint8_t 5/1 -> Mux/6  "Byte 3 will be returned here"
  uint8_t 6/1 -> Mux/7  "Byte 4 will be returned here"
  uint8_t 4/1 -> Mux/5  "Byte 2 will be returned here"
  uint8_t 8/1 -> Mux/9  "Byte 6 will be returned here"
  uint8_t 7/1 -> Mux/8  "Byte 5  will be returned here"
  uint8_t 9/1 -> Mux/10  "Byte 7 will be returned here"

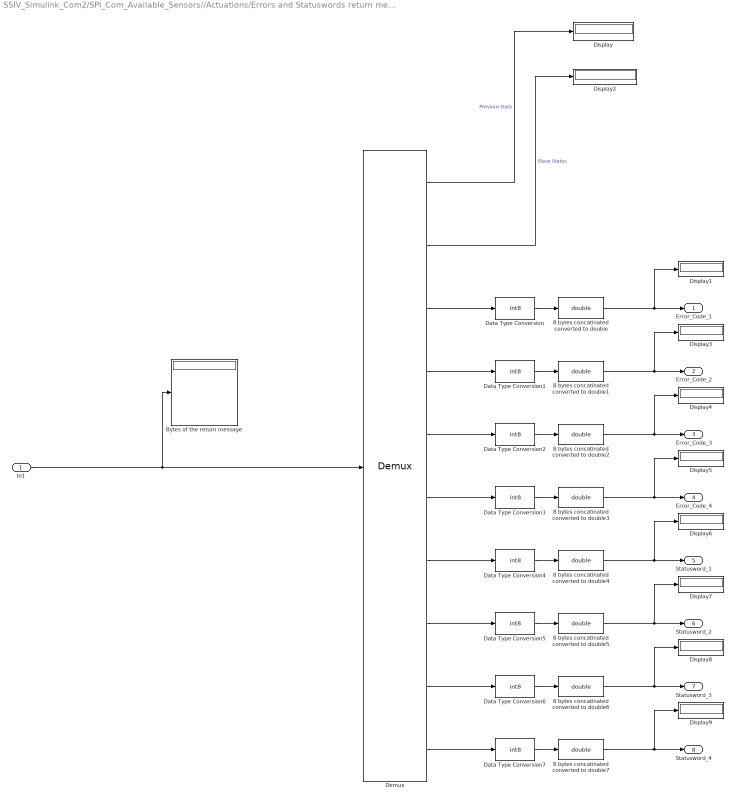
== system SSIV_Simulink_Com2/SPI_Com_Available_Sensors//Actuations/Errors and Statuswords return message (Slave --> Master) ==
  In1 : Inport
  8 bytes concatinated converted to double{,1..7} (8 alike) : DataTypeConversion  OutDataTypeStr=double  RndMeth=Nearest
  Bytes of the return message : Display
      settings: Format=decimal (Stored Integer)
  Data Type Conversion{,1..7} (8 alike) : DataTypeConversion  OutDataTypeStr=int8  RndMeth=Nearest
  Demux : Demux  Outputs=10
  Display{,1..9} (10 alike) : Display
      Display settings: Format=binary (Stored Integer)
      Display1 settings: Format=decimal (Stored Integer)
      Display2 settings: Format=binary (Stored Integer)
      Display3 settings: Format=decimal (Stored Integer)
      Display4 settings: Format=decimal (Stored Integer)
      Display5 settings: Format=decimal (Stored Integer)
      Display6 settings: Format=decimal (Stored Integer)
      Display7 settings: Format=decimal (Stored Integer)
      Display8 settings: Format=decimal (Stored Integer)
      Display9 settings: Format=decimal (Stored Integer)
  Error_Code_1 : Outport
  Error_Code_2 : Outport  Port=2
  Error_Code_3 : Outport  Port=3
  Error_Code_4 : Outport  Port=4
  Statusword_1 : Outport  Port=5
  Statusword_2 : Outport  Port=6
  Statusword_3 : Outport  Port=7
  Statusword_4 : Outport  Port=8
  wires:
  8 bytes concatinated converted to double/1 -> Display1/1, Error_Code_1/1
  Demux/1 -> Display/1  "Previous Data"
  In1/1 -> Bytes of the return message/1, Demux/1
  Data Type Conversion/1 -> 8 bytes concatinated converted to double/1
  Demux/2 -> Display2/1  "Slave Status"
  Demux/3 -> Data Type Conversion/1
  Demux/4 -> Data Type Conversion1/1
  Data Type Conversion1/1 -> 8 bytes concatinated converted to double1/1
  8 bytes concatinated converted to double1/1 -> Error_Code_2/1, Display3/1
  8 bytes concatinated converted to double2/1 -> Display4/1, Error_Code_3/1
  Data Type Conversion2/1 -> 8 bytes concatinated converted to double2/1
  Demux/5 -> Data Type Conversion2/1
  Data Type Conversion3/1 -> 8 bytes concatinated converted to double3/1
  8 bytes concatinated converted to double3/1 -> Error_Code_4/1, Display5/1
  Demux/6 -> Data Type Conversion3/1
  8 bytes concatinated converted to double4/1 -> Display6/1, Statusword_1/1
  Data Type Conversion4/1 -> 8 bytes concatinated converted to double4/1
  Demux/7 -> Data Type Conversion4/1
  Demux/8 -> Data Type Conversion5/1
  Data Type Conversion5/1 -> 8 bytes concatinated converted to double5/1
  8 bytes concatinated converted to double5/1 -> Statusword_2/1, Display7/1
  8 bytes concatinated converted to double6/1 -> Display8/1, Statusword_3/1
  Data Type Conversion6/1 -> 8 bytes concatinated converted to double6/1
  Demux/9 -> Data Type Conversion6/1
  Data Type Conversion7/1 -> 8 bytes concatinated converted to double7/1
  8 bytes concatinated converted to double7/1 -> Statusword_4/1, Display9/1
  Demux/10 -> Data Type Conversion7/1

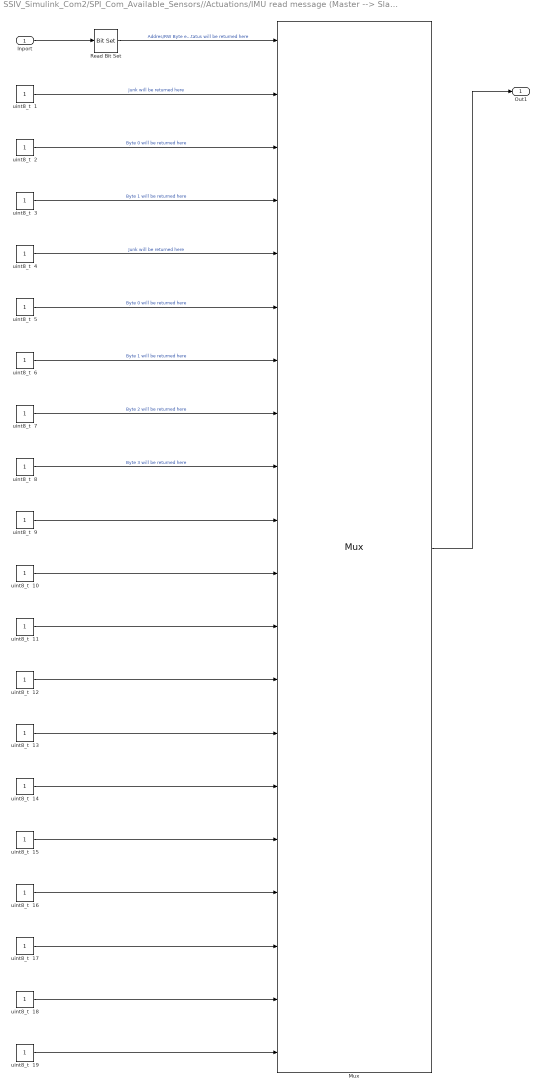
== system SSIV_Simulink_Com2/SPI_Com_Available_Sensors//Actuations/IMU read message (Master --> Slave) ==
  Inport : Inport
  Mux : Mux  Inputs=20
      settings: DisplayOption=signals
  Read Bit Set : simulink/Logic and Bit Operations/Bit Set  iBit=7
      settings: SourceProductName=Simulink  SourceProductBaseCode=SL
  uint8_t  {1..19} (19 alike) : Constant  OutDataTypeStr=uint8
  Out1 : Outport
  wires:
  Read Bit Set/1 -> Mux/1  "Addres/RW Byte euler_heading Teensy Status will be returned here"
  Inport/1 -> Read Bit Set/1
  uint8_t  3/1 -> Mux/4  "Byte 1 will be returned here"
  Mux/1 -> Out1/1
  uint8_t  2/1 -> Mux/3  "Byte 0 will be returned here"
  uint8_t  1/1 -> Mux/2  "Junk will be returned here"
  uint8_t  4/1 -> Mux/5  "Junk will be returned here"
  uint8_t  5/1 -> Mux/6  "Byte 0 will be returned here"
  uint8_t  6/1 -> Mux/7  "Byte 1 will be returned here"
  uint8_t  8/1 -> Mux/9  "Byte 3 will be returned here"
  uint8_t  7/1 -> Mux/8  "Byte 2 will be returned here"
  uint8_t  9/1 -> Mux/10
  uint8_t  16/1 -> Mux/17
  uint8_t  14/1 -> Mux/15
  uint8_t  15/1 -> Mux/16
  uint8_t  13/1 -> Mux/14
  uint8_t  12/1 -> Mux/13
  uint8_t  11/1 -> Mux/12
  uint8_t  10/1 -> Mux/11
  uint8_t  18/1 -> Mux/19
  uint8_t  17/1 -> Mux/18
  uint8_t  19/1 -> Mux/20

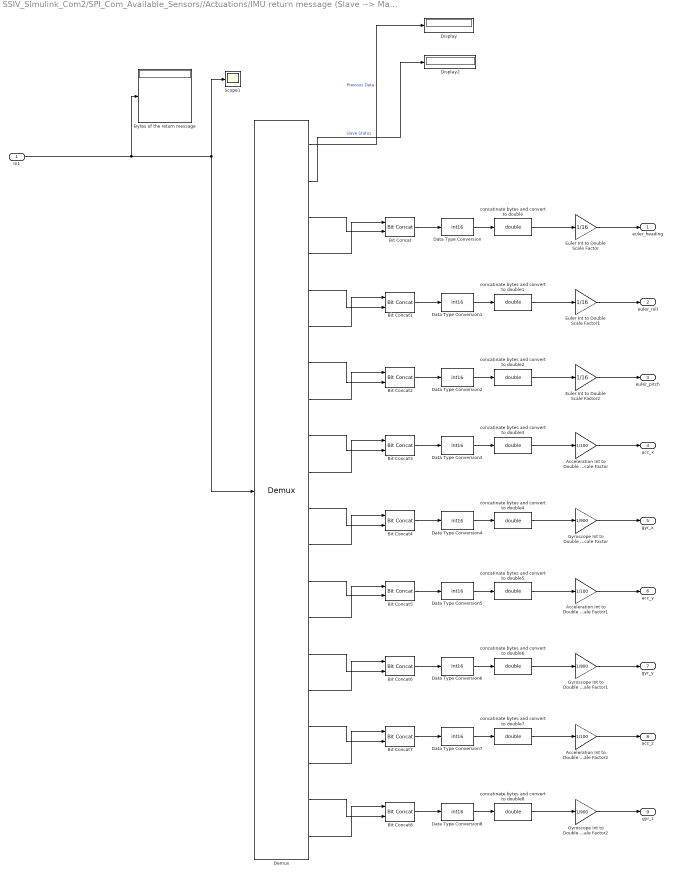
== system SSIV_Simulink_Com2/SPI_Com_Available_Sensors//Actuations/IMU return message (Slave --> Master) ==
  In1 : Inport
  Acceleration Int to Double Scale Factor : Gain  Gain=1/100
  Acceleration Int to Double Scale Factor1 : Gain  Gain=1/100
  Acceleration Int to Double Scale Factor2 : Gain  Gain=1/100
  Bit Concat{,1..8} (9 alike) : hdlsllib/Logic and Bit Operations/Bit Concat  numInputs=2
      settings: SourceProductName=HDL Coder  SourceProductBaseCode=HD
  Bytes of the return message : Display
      settings: Format=decimal (Stored Integer)
  Data Type Conversion{,1..8} (9 alike) : DataTypeConversion  OutDataTypeStr=int16  RndMeth=Nearest
  Demux : Demux  Outputs=20
  Display : Display
      settings: Format=binary (Stored Integer)
  Display2 : Display
      settings: Format=binary (Stored Integer)
  Euler Int to Double Scale Factor : Gain  Gain=1/16
  Euler Int to Double Scale Factor1 : Gain  Gain=1/16
  Euler Int to Double Scale Factor2 : Gain  Gain=1/16
  Gyroscope Int to Double Scale Factor : Gain  Gain=1/900
  Gyroscope Int to Double Scale Factor1 : Gain  Gain=1/900
  Gyroscope Int to Double Scale Factor2 : Gain  Gain=1/900
  Scope1 : Scope
  concatinate bytes and convert to double{,1..8} (9 alike) : DataTypeConversion  OutDataTypeStr=double  RndMeth=Nearest  LockScale=on
  euler_heading : Outport
  euler_roll : Outport  Port=2
  euler_pitch : Outport  Port=3
  acc_x : Outport  Port=4
  gyr_x : Outport  Port=5
  acc_y : Outport  Port=6
  gyr_y : Outport  Port=7
  acc_z : Outport  Port=8
  gyr_z : Outport  Port=9
  wires:
  concatinate bytes and convert to double/1 -> Euler Int to Double Scale Factor/1
  Demux/2 -> Display2/1  "Slave Status"
  Demux/1 -> Display/1  "Previous Data"
  In1/1 -> Bytes of the return message/1, Scope1/1, Demux/1
  Demux/4 -> Bit Concat/1
  Demux/3 -> Bit Concat/2
  Euler Int to Double Scale Factor/1 -> euler_heading/1
  Bit Concat/1 -> Data Type Conversion/1
  Data Type Conversion/1 -> concatinate bytes and convert to double/1
  Data Type Conversion1/1 -> concatinate bytes and convert to double1/1
  Bit Concat1/1 -> Data Type Conversion1/1
  Euler Int to Double Scale Factor1/1 -> euler_roll/1
  Demux/5 -> Bit Concat1/2
  Demux/6 -> Bit Concat1/1
  concatinate bytes and convert to double1/1 -> Euler Int to Double Scale Factor1/1
  concatinate bytes and convert to double2/1 -> Euler Int to Double Scale Factor2/1
  Demux/8 -> Bit Concat2/1
  Demux/7 -> Bit Concat2/2
  Euler Int to Double Scale Factor2/1 -> euler_pitch/1
  Bit Concat2/1 -> Data Type Conversion2/1
  Data Type Conversion2/1 -> concatinate bytes and convert to double2/1
  concatinate bytes and convert to double4/1 -> Gyroscope Int to Double Scale Factor/1
  Demux/12 -> Bit Concat4/1
  Demux/11 -> Bit Concat4/2
  Gyroscope Int to Double Scale Factor/1 -> gyr_x/1
  Bit Concat4/1 -> Data Type Conversion4/1
  Data Type Conversion4/1 -> concatinate bytes and convert to double4/1
  Data Type Conversion3/1 -> concatinate bytes and convert to double3/1
  Bit Concat3/1 -> Data Type Conversion3/1
  Acceleration Int to Double Scale Factor/1 -> acc_x/1
  Demux/9 -> Bit Concat3/2
  Demux/10 -> Bit Concat3/1
  concatinate bytes and convert to double3/1 -> Acceleration Int to Double Scale Factor/1
  concatinate bytes and convert to double5/1 -> Acceleration Int to Double Scale Factor1/1
  Demux/14 -> Bit Concat5/1
  Demux/13 -> Bit Concat5/2
  Acceleration Int to Double Scale Factor1/1 -> acc_y/1
  Bit Concat5/1 -> Data Type Conversion5/1
  Data Type Conversion5/1 -> concatinate bytes and convert to double5/1
  Data Type Conversion6/1 -> concatinate bytes and convert to double6/1
  Bit Concat6/1 -> Data Type Conversion6/1
  Gyroscope Int to Double Scale Factor1/1 -> gyr_y/1
  Demux/15 -> Bit Concat6/2
  Demux/16 -> Bit Concat6/1
  concatinate bytes and convert to double6/1 -> Gyroscope Int to Double Scale Factor1/1
  concatinate bytes and convert to double8/1 -> Gyroscope Int to Double Scale Factor2/1
  Demux/20 -> Bit Concat8/1
  Demux/19 -> Bit Concat8/2
  Gyroscope Int to Double Scale Factor2/1 -> gyr_z/1
  Bit Concat8/1 -> Data Type Conversion8/1
  Data Type Conversion8/1 -> concatinate bytes and convert to double8/1
  Data Type Conversion7/1 -> concatinate bytes and convert to double7/1
  Bit Concat7/1 -> Data Type Conversion7/1
  Acceleration Int to Double Scale Factor2/1 -> acc_z/1
  Demux/17 -> Bit Concat7/2
  Demux/18 -> Bit Concat7/1
  concatinate bytes and convert to double7/1 -> Acceleration Int to Double Scale Factor2/1

== system SSIV_Simulink_Com2/SPI_Com_Available_Sensors//Actuations/radio throttle and steering read message (Master --> Slave) ==
  Inport : Inport
  Mux : Mux  Inputs=6
      settings: DisplayOption=signals
  Read Bit Set : simulink/Logic and Bit Operations/Bit Set  iBit=7
      settings: SourceProductName=Simulink  SourceProductBaseCode=SL
  uint8_t {1..5} (5 alike) : Constant  OutDataTypeStr=uint8
  Out1 : Outport
  wires:
  Read Bit Set/1 -> Mux/1  "Addres/RW Byte radio_throttle Teensy Status will be returned here"
  uint8_t 1/1 -> Mux/2  "Junk will be returned here"
  Inport/1 -> Read Bit Set/1
  uint8_t 3/1 -> Mux/4  "Byte 1 will be returned here"
  Mux/1 -> Out1/1
  uint8_t 2/1 -> Mux/3  "Byte 0 will be returned here"
  uint8_t 4/1 -> Mux/5  "Byte 2 will be returned here"
  uint8_t 5/1 -> Mux/6  "Byte 3 will be returned here"

== system SSIV_Simulink_Com2/SPI_Com_Available_Sensors//Actuations/radio throttle and steering return message (Slave --> Master) ==
  In1 : Inport
  8 bytes concatinated converted to double : DataTypeConversion  OutDataTypeStr=double  RndMeth=Nearest
  8 bytes concatinated converted to double1 : DataTypeConversion  OutDataTypeStr=double  RndMeth=Nearest
  Bit Concat : hdlsllib/Logic and Bit Operations/Bit Concat  numInputs=2
      settings: SourceProductName=HDL Coder  SourceProductBaseCode=HD
  Bit Concat1 : hdlsllib/Logic and Bit Operations/Bit Concat  numInputs=2
      settings: SourceProductName=HDL Coder  SourceProductBaseCode=HD
  Bytes of the return message : Display
      settings: Format=decimal (Stored Integer)
  Data Type Conversion : DataTypeConversion  OutDataTypeStr=int16  RndMeth=Nearest
  Data Type Conversion1 : DataTypeConversion  OutDataTypeStr=int16  RndMeth=Nearest
  Demux : Demux  Outputs=6
  Display : Display
      settings: Format=binary (Stored Integer)
  Display2 : Display
      settings: Format=binary (Stored Integer)
  radio_throttle : Outport
  radio_steering : Outport  Port=2
  wires:
  8 bytes concatinated converted to double/1 -> radio_throttle/1
  Demux/2 -> Display2/1  "Slave Status"
  Demux/1 -> Display/1  "Previous Data"
  In1/1 -> Bytes of the return message/1, Demux/1
  Bit Concat/1 -> Data Type Conversion/1
  Demux/4 -> Bit Concat/1
  Demux/3 -> Bit Concat/2
  Data Type Conversion/1 -> 8 bytes concatinated converted to double/1
  Data Type Conversion1/1 -> 8 bytes concatinated converted to double1/1
  Demux/5 -> Bit Concat1/2
  Demux/6 -> Bit Concat1/1
  Bit Concat1/1 -> Data Type Conversion1/1
  8 bytes concatinated converted to double1/1 -> radio_steering/1

== system SSIV_Simulink_Com2/SPI_Com_Available_Sensors//Actuations/servo_out Write Message (Master --> Slave) ==
  In1 : Inport
  Bit Slice2 : hdlsllib/Logic and Bit Operations/Bit Slice  lidx=15  ridx=8
  Bit Slice3 : hdlsllib/Logic and Bit Operations/Bit Slice  lidx=7  ridx=0
  Display5 : Display
      settings: Format=decimal (Stored Integer)
  Mux : Mux  Inputs=2
      settings: DisplayOption=signals
  Out1 : Outport
  wires:
  In1/1 -> Display5/1, Bit Slice3/1, Bit Slice2/1  "Servo"
  Mux/1 -> Out1/1
  Bit Slice3/1 -> Mux/1
  Bit Slice2/1 -> Mux/2

== system SSIV_Simulink_Com2/SPI_Com_Available_Sensors//Actuations/torque Write Message (Master --> Slave) ==
  In1 : Inport
  In2 : Inport  Port=2
  In3 : Inport  Port=3
  In4 : Inport  Port=4
  Bit Slice{,2,4,6} (4 alike) : hdlsllib/Logic and Bit Operations/Bit Slice  lidx=15  ridx=8
  Bit Slice{1,3,5,7} (4 alike) : hdlsllib/Logic and Bit Operations/Bit Slice  lidx=7  ridx=0
  Mux : Mux  Inputs=8
      settings: DisplayOption=signals
  Output : Outport
  wires:
  Bit Slice/1 -> Mux/2
  Bit Slice1/1 -> Mux/1
  In1/1 -> Bit Slice/1, Bit Slice1/1
  In2/1 -> Bit Slice3/1, Bit Slice2/1
  Bit Slice3/1 -> Mux/3
  Bit Slice2/1 -> Mux/4
  Bit Slice4/1 -> Mux/6
  Bit Slice5/1 -> Mux/5
  In3/1 -> Bit Slice4/1, Bit Slice5/1
  In4/1 -> Bit Slice7/1, Bit Slice6/1
  Bit Slice7/1 -> Mux/7
  Bit Slice6/1 -> Mux/8
  Mux/1 -> Output/1
